simulink model "W01_Base_Map_cs"  (R2019a)
(part 2 of 32)

      settings: OpenFcn=open_system([gcb '/Actuator'],'mask')
      mask Help: eval('openHelp(230)')
      mask Display: image(imread('TextureColor.png'))
  VISUColorRegion_Lower_Body_Male_wLongCoat_1 : Subsystem  Tag=actuator/ColorRegion  Priority=0  LoadFcn=load('PrescanColorData')  mask(PreScan Sink Block: VisuTextureColor){}
      mask help:
      | The VisuTextureColor block provides a way to adapt the color of a vehicle.
      |
      | For more information, please click Help.
      settings: OpenFcn=open_system([gcb '/Actuator'],'mask')
      mask Help: eval('openHelp(230)')
      mask Display: image(imread('TextureColor.png'))
  VISUColorRegion_Lower_Body_Man_250_1 : Subsystem  Tag=actuator/ColorRegion  Priority=0  LoadFcn=load('PrescanColorData')  mask(PreScan Sink Block: VisuTextureColor){}
      mask help:
      | The VisuTextureColor block provides a way to adapt the color of a vehicle.
      |
      | For more information, please click Help.
      settings: OpenFcn=open_system([gcb '/Actuator'],'mask')
      mask Help: eval('openHelp(230)')
      mask Display: image(imread('TextureColor.png'))
  VISUColorRegion_Shoes_Boy_150_1 : Subsystem  Tag=actuator/ColorRegion  Priority=0  LoadFcn=load('PrescanColorData')  mask(PreScan Sink Block: VisuTextureColor){}
      mask help:
      | The VisuTextureColor block provides a way to adapt the color of a vehicle.
      |
      | For more information, please click Help.
      settings: OpenFcn=open_system([gcb '/Actuator'],'mask')
      mask Help: eval('openHelp(230)')
      mask Display: image(imread('TextureColor.png'))
  VISUColorRegion_Shoes_Child_Overweight_1 : Subsystem  Tag=actuator/ColorRegion  Priority=0  LoadFcn=load('PrescanColorData')  mask(PreScan Sink Block: VisuTextureColor){}
      mask help:
      | The VisuTextureColor block provides a way to adapt the color of a vehicle.
      |
      | For more information, please click Help.
      settings: OpenFcn=open_system([gcb '/Actuator'],'mask')
      mask Help: eval('openHelp(230)')
      mask Display: image(imread('TextureColor.png'))
  VISUColorRegion_Shoes_Female_Overweight_1 : Subsystem  Tag=actuator/ColorRegion  Priority=0  LoadFcn=load('PrescanColorData')  mask(PreScan Sink Block: VisuTextureColor){}
      mask help:
      | The VisuTextureColor block provides a way to adapt the color of a vehicle.
      |
      | For more information, please click Help.
      settings: OpenFcn=open_system([gcb '/Actuator'],'mask')
      mask Help: eval('openHelp(230)')
      mask Display: image(imread('TextureColor.png'))
  VISUColorRegion_Shoes_Female_Regular_1 : Subsystem  Tag=actuator/ColorRegion  Priority=0  LoadFcn=load('PrescanColorData')  mask(PreScan Sink Block: VisuTextureColor){}
      mask help:
      | The VisuTextureColor block provides a way to adapt the color of a vehicle.
      |
      | For more information, please click Help.
      settings: OpenFcn=open_system([gcb '/Actuator'],'mask')
      mask Help: eval('openHelp(230)')
      mask Display: image(imread('TextureColor.png'))
  VISUColorRegion_Shoes_Female_wBuggy_1 : Subsystem  Tag=actuator/ColorRegion  Priority=0  LoadFcn=load('PrescanColorData')  mask(PreScan Sink Block: VisuTextureColor){}
      mask help:
      | The VisuTextureColor block provides a way to adapt the color of a vehicle.
      |
      | For more information, please click Help.
      settings: OpenFcn=open_system([gcb '/Actuator'],'mask')
      mask Help: eval('openHelp(230)')
      mask Display: image(imread('TextureColor.png'))
  VISUColorRegion_Shoes_Female_wLongCoat_1 : Subsystem  Tag=actuator/ColorRegion  Priority=0  LoadFcn=load('PrescanColorData')  mask(PreScan Sink Block: VisuTextureColor){}
      mask help:
      | The VisuTextureColor block provides a way to adapt the color of a vehicle.
      |
      | For more information, please click Help.
      settings: OpenFcn=open_system([gcb '/Actuator'],'mask')
      mask Help: eval('openHelp(230)')
      mask Display: image(imread('TextureColor.png'))
  VISUColorRegion_Shoes_Female_wRaincoat_1 : Subsystem  Tag=actuator/ColorRegion  Priority=0  LoadFcn=load('PrescanColorData')  mask(PreScan Sink Block: VisuTextureColor){}
      mask help:
      | The VisuTextureColor block provides a way to adapt the color of a vehicle.
      |
      | For more information, please click Help.
      settings: OpenFcn=open_system([gcb '/Actuator'],'mask')
      mask Help: eval('openHelp(230)')
      mask Display: image(imread('TextureColor.png'))
  VISUColorRegion_Shoes_Male_200_1 : Subsystem  Tag=actuator/ColorRegion  Priority=0  LoadFcn=load('PrescanColorData')  mask(PreScan Sink Block: VisuTextureColor){}
      mask help:
      | The VisuTextureColor block provides a way to adapt the color of a vehicle.
      |
      | For more information, please click Help.
      settings: OpenFcn=open_system([gcb '/Actuator'],'mask')
      mask Help: eval('openHelp(230)')
      mask Display: image(imread('TextureColor.png'))
  VISUColorRegion_Shoes_Male_African_1 : Subsystem  Tag=actuator/ColorRegion  Priority=0  LoadFcn=load('PrescanColorData')  mask(PreScan Sink Block: VisuTextureColor){}
      mask help:
      | The VisuTextureColor block provides a way to adapt the color of a vehicle.
      |
      | For more information, please click Help.
      settings: OpenFcn=open_system([gcb '/Actuator'],'mask')
      mask Help: eval('openHelp(230)')
      mask Display: image(imread('TextureColor.png'))
  VISUColorRegion_Shoes_Male_LargeShoulderSuitcase_1 : Subsystem  Tag=actuator/ColorRegion  Priority=0  LoadFcn=load('PrescanColorData')  mask(PreScan Sink Block: VisuTextureColor){}
      mask help:
      | The VisuTextureColor block provides a way to adapt the color of a vehicle.
      |
      | For more information, please click Help.
      settings: OpenFcn=open_system([gcb '/Actuator'],'mask')
      mask Help: eval('openHelp(230)')
      mask Display: image(imread('TextureColor.png'))
  VISUColorRegion_Shoes_Male_Old_White_WithStick_1 : Subsystem  Tag=actuator/ColorRegion  Priority=0  LoadFcn=load('PrescanColorData')  mask(PreScan Sink Block: VisuTextureColor){}
      mask help:
      | The VisuTextureColor block provides a way to adapt the color of a vehicle.
      |
      | For more information, please click Help.
      settings: OpenFcn=open_system([gcb '/Actuator'],'mask')
      mask Help: eval('openHelp(230)')
      mask Display: image(imread('TextureColor.png'))
  VISUColorRegion_Shoes_Male_Old_White_WithWalkerWithWheels_1 : Subsystem  Tag=actuator/ColorRegion  Priority=0  LoadFcn=load('PrescanColorData')  mask(PreScan Sink Block: VisuTextureColor){}
      mask help:
      | The VisuTextureColor block provides a way to adapt the color of a vehicle.
      |
      | For more information, please click Help.
      settings: OpenFcn=open_system([gcb '/Actuator'],'mask')
      mask Help: eval('openHelp(230)')
      mask Display: image(imread('TextureColor.png'))
  VISUColorRegion_Shoes_Male_Overweight_1 : Subsystem  Tag=actuator/ColorRegion  Priority=0  LoadFcn=load('PrescanColorData')  mask(PreScan Sink Block: VisuTextureColor){}
      mask help:
      | The VisuTextureColor block provides a way to adapt the color of a vehicle.
      |
      | For more information, please click Help.
      settings: OpenFcn=open_system([gcb '/Actuator'],'mask')
      mask Help: eval('openHelp(230)')
      mask Display: image(imread('TextureColor.png'))
  VISUColorRegion_Shoes_Male_ShoppingBag_1 : Subsystem  Tag=actuator/ColorRegion  Priority=0  LoadFcn=load('PrescanColorData')  mask(PreScan Sink Block: VisuTextureColor){}
      mask help:
      | The VisuTextureColor block provides a way to adapt the color of a vehicle.
      |
      | For more information, please click Help.
      settings: OpenFcn=open_system([gcb '/Actuator'],'mask')
      mask Help: eval('openHelp(230)')
      mask Display: image(imread('TextureColor.png'))
  VISUColorRegion_Shoes_Male_wBackpack_1 : Subsystem  Tag=actuator/ColorRegion  Priority=0  LoadFcn=load('PrescanColorData')  mask(PreScan Sink Block: VisuTextureColor){}
      mask help:
      | The VisuTextureColor block provides a way to adapt the color of a vehicle.
      |
      | For more information, please click Help.
      settings: OpenFcn=open_system([gcb '/Actuator'],'mask')
      mask Help: eval('openHelp(230)')
      mask Display: image(imread('TextureColor.png'))
  VISUColorRegion_Shoes_Male_wLargeBackpack_1 : Subsystem  Tag=actuator/ColorRegion  Priority=0  LoadFcn=load('PrescanColorData')  mask(PreScan Sink Block: VisuTextureColor){}
      mask help:
      | The VisuTextureColor block provides a way to adapt the color of a vehicle.
      |
      | For more information, please click Help.
      settings: OpenFcn=open_system([gcb '/Actuator'],'mask')
      mask Help: eval('openHelp(230)')
      mask Display: image(imread('TextureColor.png'))
  VISUColorRegion_Shoes_Male_wLongCoat_1 : Subsystem  Tag=actuator/ColorRegion  Priority=0  LoadFcn=load('PrescanColorData')  mask(PreScan Sink Block: VisuTextureColor){}
      mask help:
      | The VisuTextureColor block provides a way to adapt the color of a vehicle.
      |
      | For more information, please click Help.
      settings: OpenFcn=open_system([gcb '/Actuator'],'mask')
      mask Help: eval('openHelp(230)')
      mask Display: image(imread('TextureColor.png'))
  VISUColorRegion_Shoes_Man_250_1 : Subsystem  Tag=actuator/ColorRegion  Priority=0  LoadFcn=load('PrescanColorData')  mask(PreScan Sink Block: VisuTextureColor){}
      mask help:
      | The VisuTextureColor block provides a way to adapt the color of a vehicle.
      |
      | For more information, please click Help.
      settings: OpenFcn=open_system([gcb '/Actuator'],'mask')
      mask Help: eval('openHelp(230)')
      mask Display: image(imread('TextureColor.png'))
  VISUColorRegion_Upper_Body_Boy_150_1 : Subsystem  Tag=actuator/ColorRegion  Priority=0  LoadFcn=load('PrescanColorData')  mask(PreScan Sink Block: VisuTextureColor){}
      mask help:
      | The VisuTextureColor block provides a way to adapt the color of a vehicle.
      |
      | For more information, please click Help.
      settings: OpenFcn=open_system([gcb '/Actuator'],'mask')
      mask Help: eval('openHelp(230)')
      mask Display: image(imread('TextureColor.png'))
  VISUColorRegion_Upper_Body_Child_Overweight_1 : Subsystem  Tag=actuator/ColorRegion  Priority=0  LoadFcn=load('PrescanColorData')  mask(PreScan Sink Block: VisuTextureColor){}
      mask help:
      | The VisuTextureColor block provides a way to adapt the color of a vehicle.
      |
      | For more information, please click Help.
      settings: OpenFcn=open_system([gcb '/Actuator'],'mask')
      mask Help: eval('openHelp(230)')
      mask Display: image(imread('TextureColor.png'))
  VISUColorRegion_Upper_Body_Female_Overweight_1 : Subsystem  Tag=actuator/ColorRegion  Priority=0  LoadFcn=load('PrescanColorData')  mask(PreScan Sink Block: VisuTextureColor){}
      mask help:
      | The VisuTextureColor block provides a way to adapt the color of a vehicle.
      |
      | For more information, please click Help.
      settings: OpenFcn=open_system([gcb '/Actuator'],'mask')
      mask Help: eval('openHelp(230)')
      mask Display: image(imread('TextureColor.png'))
  VISUColorRegion_Upper_Body_Female_Regular_1 : Subsystem  Tag=actuator/ColorRegion  Priority=0  LoadFcn=load('PrescanColorData')  mask(PreScan Sink Block: VisuTextureColor){}
      mask help:
      | The VisuTextureColor block provides a way to adapt the color of a vehicle.
      |
      | For more information, please click Help.
      settings: OpenFcn=open_system([gcb '/Actuator'],'mask')
      mask Help: eval('openHelp(230)')
      mask Display: image(imread('TextureColor.png'))
  VISUColorRegion_Upper_Body_Female_wBuggy_1 : Subsystem  Tag=actuator/ColorRegion  Priority=0  LoadFcn=load('PrescanColorData')  mask(PreScan Sink Block: VisuTextureColor){}
      mask help:
      | The VisuTextureColor block provides a way to adapt the color of a vehicle.
      |
      | For more information, please click Help.
      settings: OpenFcn=open_system([gcb '/Actuator'],'mask')
      mask Help: eval('openHelp(230)')
      mask Display: image(imread('TextureColor.png'))
  VISUColorRegion_Upper_Body_Female_wLongCoat_1 : Subsystem  Tag=actuator/ColorRegion  Priority=0  LoadFcn=load('PrescanColorData')  mask(PreScan Sink Block: VisuTextureColor){}
      mask help:
      | The VisuTextureColor block provides a way to adapt the color of a vehicle.
      |
      | For more information, please click Help.
      settings: OpenFcn=open_system([gcb '/Actuator'],'mask')
      mask Help: eval('openHelp(230)')
      mask Display: image(imread('TextureColor.png'))
  VISUColorRegion_Upper_Body_Female_wRaincoat_1 : Subsystem  Tag=actuator/ColorRegion  Priority=0  LoadFcn=load('PrescanColorData')  mask(PreScan Sink Block: VisuTextureColor){}
      mask help:
      | The VisuTextureColor block provides a way to adapt the color of a vehicle.
      |
      | For more information, please click Help.
      settings: OpenFcn=open_system([gcb '/Actuator'],'mask')
      mask Help: eval('openHelp(230)')
      mask Display: image(imread('TextureColor.png'))
  VISUColorRegion_Upper_Body_Male_200_1 : Subsystem  Tag=actuator/ColorRegion  Priority=0  LoadFcn=load('PrescanColorData')  mask(PreScan Sink Block: VisuTextureColor){}
      mask help:
      | The VisuTextureColor block provides a way to adapt the color of a vehicle.
      |
      | For more information, please click Help.
      settings: OpenFcn=open_system([gcb '/Actuator'],'mask')
      mask Help: eval('openHelp(230)')
      mask Display: image(imread('TextureColor.png'))
  VISUColorRegion_Upper_Body_Male_African_1 : Subsystem  Tag=actuator/ColorRegion  Priority=0  LoadFcn=load('PrescanColorData')  mask(PreScan Sink Block: VisuTextureColor){}
      mask help:
      | The VisuTextureColor block provides a way to adapt the color of a vehicle.
      |
      | For more information, please click Help.
      settings: OpenFcn=open_system([gcb '/Actuator'],'mask')
      mask Help: eval('openHelp(230)')
      mask Display: image(imread('TextureColor.png'))
  VISUColorRegion_Upper_Body_Male_Old_White_WithStick_1 : Subsystem  Tag=actuator/ColorRegion  Priority=0  LoadFcn=load('PrescanColorData')  mask(PreScan Sink Block: VisuTextureColor){}
      mask help:
      | The VisuTextureColor block provides a way to adapt the color of a vehicle.
      |
      | For more information, please click Help.
      settings: OpenFcn=open_system([gcb '/Actuator'],'mask')
      mask Help: eval('openHelp(230)')
      mask Display: image(imread('TextureColor.png'))
  VISUColorRegion_Upper_Body_Male_Old_White_WithWalkerWithWheels_1 : Subsystem  Tag=actuator/ColorRegion  Priority=0  LoadFcn=load('PrescanColorData')  mask(PreScan Sink Block: VisuTextureColor){}
      mask help:
      | The VisuTextureColor block provides a way to adapt the color of a vehicle.
      |
      | For more information, please click Help.
      settings: OpenFcn=open_system([gcb '/Actuator'],'mask')
      mask Help: eval('openHelp(230)')
      mask Display: image(imread('TextureColor.png'))
  VISUColorRegion_Upper_Body_Male_ShoppingBag_1 : Subsystem  Tag=actuator/ColorRegion  Priority=0  LoadFcn=load('PrescanColorData')  mask(PreScan Sink Block: VisuTextureColor){}
      mask help:
      | The VisuTextureColor block provides a way to adapt the color of a vehicle.
      |
      | For more information, please click Help.
      settings: OpenFcn=open_system([gcb '/Actuator'],'mask')
      mask Help: eval('openHelp(230)')
      mask Display: image(imread('TextureColor.png'))
  VISUColorRegion_Upper_Body_Male_wBackpack_1 : Subsystem  Tag=actuator/ColorRegion  Priority=0  LoadFcn=load('PrescanColorData')  mask(PreScan Sink Block: VisuTextureColor){}
      mask help:
      | The VisuTextureColor block provides a way to adapt the color of a vehicle.
      |
      | For more information, please click Help.
      settings: OpenFcn=open_system([gcb '/Actuator'],'mask')
      mask Help: eval('openHelp(230)')
      mask Display: image(imread('TextureColor.png'))
  VISUColorRegion_Upper_Body_Male_wLongCoat_1 : Subsystem  Tag=actuator/ColorRegion  Priority=0  LoadFcn=load('PrescanColorData')  mask(PreScan Sink Block: VisuTextureColor){}
      mask help:
      | The VisuTextureColor block provides a way to adapt the color of a vehicle.
      |
      | For more information, please click Help.
      settings: OpenFcn=open_system([gcb '/Actuator'],'mask')
      mask Help: eval('openHelp(230)')
      mask Display: image(imread('TextureColor.png'))
  VISUColorRegion_Upper_Body_Man_250_1 : Subsystem  Tag=actuator/ColorRegion  Priority=0  LoadFcn=load('PrescanColorData')  mask(PreScan Sink Block: VisuTextureColor){}
      mask help:
      | The VisuTextureColor block provides a way to adapt the color of a vehicle.
      |
      | For more information, please click Help.
      settings: OpenFcn=open_system([gcb '/Actuator'],'mask')
      mask Help: eval('openHelp(230)')
      mask Display: image(imread('TextureColor.png'))
  VISUColorRegion_Upper_body_Male_LargeShoulderSuitcase_1 : Subsystem  Tag=actuator/ColorRegion  Priority=0  LoadFcn=load('PrescanColorData')  mask(PreScan Sink Block: VisuTextureColor){}
      mask help:
      | The VisuTextureColor block provides a way to adapt the color of a vehicle.
      |
      | For more information, please click Help.
      settings: OpenFcn=open_system([gcb '/Actuator'],'mask')
      mask Help: eval('openHelp(230)')
      mask Display: image(imread('TextureColor.png'))
  VISUColorRegion_Upper_body_Male_wLargeBackpack_1 : Subsystem  Tag=actuator/ColorRegion  Priority=0  LoadFcn=load('PrescanColorData')  mask(PreScan Sink Block: VisuTextureColor){}
      mask help:
      | The VisuTextureColor block provides a way to adapt the color of a vehicle.
      |
      | For more information, please click Help.
      settings: OpenFcn=open_system([gcb '/Actuator'],'mask')
      mask Help: eval('openHelp(230)')
      mask Display: image(imread('TextureColor.png'))
  Vector Concatenate : Concatenate  Commented=on  NumInputs=3
  Volvo_XC60_1 : Subsystem  Tag=WorldObjectSubSystem  InitFcn=UniqueId = '29038';
      mask init:
      | modelPath = GenericModelHelper.getGenericModelFilePath('ModelDepo','Vehicles\Volvo_XC60\VolvoXC60.pgmb','fe213b90741b40e4bc1c1ba1f9c63fa4');imagePath = GenericModelHelper.getCompilationPicture(modelPath, 'Volvo_XC60.png');
      mask Display: image(imread(imagePath));color('white');text(0, 0, ' ID=122\n')
  Wuling_Hongguang_1 : Subsystem  Tag=WorldObjectSubSystem  InitFcn=UniqueId = '29075';
      mask init:
      | modelPath = GenericModelHelper.getGenericModelFilePath('ModelDepo','Vehicles\Wuling_Hongguang\Wuling_Hongguang.pgmb','c2d1d1bd61267082ac42dab8ff861914');imagePath = GenericModelHelper.getCompilationPicture(modelPath, 'Wuling_Hongguang.png');
      mask Display: image(imread(imagePath));color('white');text(0, 0, ' ID=151\n')
  pose_otheCar : Subsystem  Commented=on
  wires:
  From9/1 -> pose_otheCar/Enable
  Vector Concatenate/1 -> pose_otheCar/1(In1)
  Subsystem/1(Out1) -> Female_Regular_1/2(In1)
  Subsystem/2(Out2) -> Male_wLargeBackpack_1/2(In1)
  Subsystem/3(Out3) -> Male_wBackpack_1/2(In1)
  Subsystem/4(Out4) -> Male_ShoppingBag_1/2(In1)
  Subsystem/5(Out5) -> Male_LargeShoulderSuitcase_1/2(In1)
  Subsystem/6(Out6) -> Male_wLongCoat_1/2(In1)
  Subsystem/7(Out7) -> Honda_Pan_European_Motorcycle_With_Driver_1/2(In1)
  Subsystem/8(Out8) -> Sports_Bike_wDriver_1/2(In1)
  Subsystem/9(Out9) -> Tesla_Model_3_1/2(In1)
  Subsystem/10(Out10) -> Volvo_XC60_1/2(In1)
  Subsystem/11(Out11) -> Boy_150_1/2(In1)
  Subsystem/12(Out12) -> Child_Overweight_1/2(In1)
  Subsystem/13(Out13) -> Female_Overweight_1/2(In1)
  Subsystem/14(Out14) -> Female_wBuggy_1/2(In1)
  Subsystem/15(Out15) -> Female_wLongCoat_1/2(In1)
  Subsystem/16(Out16) -> Female_wRaincoat_1/2(In1)
  Subsystem/17(Out17) -> Male_African_1/2(In1)
  Subsystem/18(Out18) -> Male_Old_White_WithStick_1/2(In1)
  Subsystem/19(Out19) -> Male_Overweight_1/2(In1)
  Subsystem/20(Out20) -> Male_wSuit_1/2(In1)
  Subsystem/21(Out21) -> Male_200_1/2(In1)
  Subsystem/22(Out22) -> Man_250_1/2(In1)
  Subsystem/23(Out23) -> Male_Old_White_WithWalker_1/2(In1)
  Subsystem/24(Out24) -> Male_Old_White_WithWalkerWithWheels_1/2(In1)
  Subsystem/25(Out25) -> Audi_A3_1/2(In1)
  Subsystem/26(Out26) -> Audi_A8_Sedan_2/2(In1)
  Subsystem/27(Out27) -> BMW_Z3_Convertible_1/2(In1)
  Subsystem/28(Out28) -> Citroen_C3_Hatchback_2/2(In1)
  Subsystem/29(Out29) -> Fiat_Bravo_Hatchback_1/2(In1)
  Subsystem/30(Out30) -> Ford_Fiesta_Hatchback_2/2(In1)
  Subsystem/31(Out31) -> Ford_Focus_Stationwagon_1/2(In1)
  Subsystem/32(Out32) -> Lexus_GS_450h_F_Sport_Sedan_1/2(In1)
  Subsystem/33(Out33) -> Lexus_LS_600h_F_Sport_1/2(In1)
  Subsystem/34(Out34) -> Mazda_RX8_Coupe_1/2(In1)
  Subsystem/35(Out35) -> Roewe_550_S_Sedan_1/2(In1)
  Subsystem/36(Out36) -> Toyota_Previa_MPV_1/2(In1)
  Subsystem/37(Out37) -> Toyota_Prius_Sedan_1/2(In1)
  Subsystem/38(Out38) -> Toyota_Yaris_Hatchback_1/2(In1)
  Subsystem/39(Out39) -> Wuling_Hongguang_1/2(In1)
  Subsystem/40(Out40) -> Toyota_Yaris_Hatchback_2/2(In1)
  Subsystem/41(Out41) -> Citroen_C3_Hatchback_3/2(In1)
  Subsystem/42(Out42) -> Audi_A3_2/2(In1)
  Subsystem/43(Out43) -> Sports_Bike_wDriver_2/2(In1)
  Subsystem/44(Out44) -> Sports_Bike_wDriver_3/2(In1)
  Subsystem/45(Out45) -> Honda_Pan_European_Motorcycle_With_Driver_2/2(In1)
  Subsystem/46(Out46) -> Male_CyclingCyclist_1/2(In1)
  Subsystem/47(Out47) -> Male_CyclingCyclist_2/2(In1)
  Subsystem/48(Out48) -> Male_CyclingCyclist_3/2(In1)
  Subsystem/49(Out49) -> Male_CyclingCyclist_4/2(In1)
  Subsystem/50(Out50) -> Male_CyclingCyclist_5/2(In1)
  Subsystem/51(Out51) -> Male_CyclingCyclist_6/2(In1)
  Subsystem/52(Out52) -> Male_CyclingCyclist_7/2(In1)
  Subsystem/53(Out53) -> Male_CyclingCyclist_8/2(In1)
  Subsystem/54(Out54) -> Male_CyclingCyclist_9/2(In1)
  Subsystem/55(Out55) -> Male_CyclingCyclist_10/2(In1)
  BMW_X5_SUV_1/1(STATE_BMW_X5_SUV_1_bus) -> STATE_BMW_X5_SUV_1_bus/1(STATE_BMW_X5_SUV_1_bus)
  SELF_BMW_X5_SUV_1/1(SELF_BMW_X5_SUV_1) -> BMW_X5_SUV_1/1(SELF_BMW_X5_SUV_1)
  Radar_1/1(Radar_1) -> BMW_X5_SUV_1/2(Radar_1)
  PointCloudSensor_1/1(PointCloudSensor_1) -> BMW_X5_SUV_1/3(PointCloudSensor_1)
  PointCloudSensor_2/1(PointCloudSensor_2) -> BMW_X5_SUV_1/4(PointCloudSensor_2)
  PointCloudSensor_3/1(PointCloudSensor_3) -> BMW_X5_SUV_1/5(PointCloudSensor_3)
  PointCloudSensor_4/1(PointCloudSensor_4) -> BMW_X5_SUV_1/6(PointCloudSensor_4)
  Camera_1/1(Camera_1) -> BMW_X5_SUV_1/7(Camera_1)
  Camera_tl/1(Camera_tl) -> BMW_X5_SUV_1/8(Camera_tl)
  Camera_2/1(Camera_2) -> BMW_X5_SUV_1/9(Camera_2)
  TrafficLightRoadSideNL_1/1(TrafficLightRoadSideNL_1_Red) -> TrafficLightRoadSideNL_1_Red/1(TrafficLightRoadSideNL_1_Red)
  TrafficLightRoadSideNL_1/2(TrafficLightRoadSideNL_1_Orange) -> TrafficLightRoadSideNL_1_Orange/1(TrafficLightRoadSideNL_1_Orange)
  TrafficLightRoadSideNL_1/3(TrafficLightRoadSideNL_1_Green) -> TrafficLightRoadSideNL_1_Green/1(TrafficLightRoadSideNL_1_Green)
  TrafficLightRoadSideNL_2/1(TrafficLightRoadSideNL_2_Red) -> TrafficLightRoadSideNL_2_Red/1(TrafficLightRoadSideNL_2_Red)
  TrafficLightRoadSideNL_2/2(TrafficLightRoadSideNL_2_Orange) -> TrafficLightRoadSideNL_2_Orange/1(TrafficLightRoadSideNL_2_Orange)
  TrafficLightRoadSideNL_2/3(TrafficLightRoadSideNL_2_Green) -> TrafficLightRoadSideNL_2_Green/1(TrafficLightRoadSideNL_2_Green)
  TrafficLightRoadSideNL_3/1(TrafficLightRoadSideNL_3_Red) -> TrafficLightRoadSideNL_3_Red/1(TrafficLightRoadSideNL_3_Red)
  TrafficLightRoadSideNL_3/2(TrafficLightRoadSideNL_3_Orange) -> TrafficLightRoadSideNL_3_Orange/1(TrafficLightRoadSideNL_3_Orange)
  TrafficLightRoadSideNL_3/3(TrafficLightRoadSideNL_3_Green) -> TrafficLightRoadSideNL_3_Green/1(TrafficLightRoadSideNL_3_Green)
  TrafficLightRoadSideNL_4/1(TrafficLightRoadSideNL_4_Red) -> TrafficLightRoadSideNL_4_Red/1(TrafficLightRoadSideNL_4_Red)
  TrafficLightRoadSideNL_4/2(TrafficLightRoadSideNL_4_Orange) -> TrafficLightRoadSideNL_4_Orange/1(TrafficLightRoadSideNL_4_Orange)
  TrafficLightRoadSideNL_4/3(TrafficLightRoadSideNL_4_Green) -> TrafficLightRoadSideNL_4_Green/1(TrafficLightRoadSideNL_4_Green)
  TrafficLightRoadSideNL_5/1(TrafficLightRoadSideNL_5_Red) -> TrafficLightRoadSideNL_5_Red/1(TrafficLightRoadSideNL_5_Red)
  TrafficLightRoadSideNL_5/2(TrafficLightRoadSideNL_5_Orange) -> TrafficLightRoadSideNL_5_Orange/1(TrafficLightRoadSideNL_5_Orange)
  TrafficLightRoadSideNL_5/3(TrafficLightRoadSideNL_5_Green) -> TrafficLightRoadSideNL_5_Green/1(TrafficLightRoadSideNL_5_Green)
  TrafficLightRoadSideNL_7/1(TrafficLightRoadSideNL_7_Red) -> TrafficLightRoadSideNL_7_Red/1(TrafficLightRoadSideNL_7_Red)
  TrafficLightRoadSideNL_7/2(TrafficLightRoadSideNL_7_Orange) -> TrafficLightRoadSideNL_7_Orange/1(TrafficLightRoadSideNL_7_Orange)
  TrafficLightRoadSideNL_7/3(TrafficLightRoadSideNL_7_Green) -> TrafficLightRoadSideNL_7_Green/1(TrafficLightRoadSideNL_7_Green)
  TrafficLightRoadSideNL_8/1(TrafficLightRoadSideNL_8_Red) -> TrafficLightRoadSideNL_8_Red/1(TrafficLightRoadSideNL_8_Red)
  TrafficLightRoadSideNL_8/2(TrafficLightRoadSideNL_8_Orange) -> TrafficLightRoadSideNL_8_Orange/1(TrafficLightRoadSideNL_8_Orange)
  TrafficLightRoadSideNL_8/3(TrafficLightRoadSideNL_8_Green) -> TrafficLightRoadSideNL_8_Green/1(TrafficLightRoadSideNL_8_Green)
  TrafficLightRoadSideNL_6/1(TrafficLightRoadSideNL_6_Red) -> TrafficLightRoadSideNL_6_Red/1(TrafficLightRoadSideNL_6_Red)
  TrafficLightRoadSideNL_6/2(TrafficLightRoadSideNL_6_Orange) -> TrafficLightRoadSideNL_6_Orange/1(TrafficLightRoadSideNL_6_Orange)
  TrafficLightRoadSideNL_6/3(TrafficLightRoadSideNL_6_Green) -> TrafficLightRoadSideNL_6_Green/1(TrafficLightRoadSideNL_6_Green)
  Female_Regular_1/1(STATE_Female_Regular_1_bus) -> STATE_Female_Regular_1_bus/1(STATE_Female_Regular_1_bus)
  Female_Regular_1/2(ANIM_Female_Regular_1) -> ANIM_Female_Regular_1/1(ANIM_Female_Regular_1)
  SELF_Female_Regular_1/1(SELF_Female_Regular_1) -> Female_Regular_1/1(SELF_Female_Regular_1)
  Female_Regular_1/3(VISUColorRegion_Upper_Body_Female_Regular_1) -> VISUColorRegion_Upper_Body_Female_Regular_1/1(VISUColorRegion_Upper_Body_Female_Regular_1)
  Female_Regular_1/4(VISUColorRegion_Lower_Body_Female_Regular_1) -> VISUColorRegion_Lower_Body_Female_Regular_1/1(VISUColorRegion_Lower_Body_Female_Regular_1)
  Female_Regular_1/5(VISUColorRegion_Shoes_Female_Regular_1) -> VISUColorRegion_Shoes_Female_Regular_1/1(VISUColorRegion_Shoes_Female_Regular_1)
  Male_wLargeBackpack_1/1(STATE_Male_wLargeBackpack_1_bus) -> STATE_Male_wLargeBackpack_1_bus/1(STATE_Male_wLargeBackpack_1_bus)
  Male_wLargeBackpack_1/2(ANIM_Male_wLargeBackpack_1) -> ANIM_Male_wLargeBackpack_1/1(ANIM_Male_wLargeBackpack_1)
  SELF_Male_wLargeBackpack_1/1(SELF_Male_wLargeBackpack_1) -> Male_wLargeBackpack_1/1(SELF_Male_wLargeBackpack_1)
  Male_wLargeBackpack_1/3(VISUColorRegion_Upper_body_Male_wLargeBackpack_1) -> VISUColorRegion_Upper_body_Male_wLargeBackpack_1/1(VISUColorRegion_Upper_body_Male_wLargeBackpack_1)
  Male_wLargeBackpack_1/4(VISUColorRegion_Lower_Body_Male_wLargeBackpack_1) -> VISUColorRegion_Lower_Body_Male_wLargeBackpack_1/1(VISUColorRegion_Lower_Body_Male_wLargeBackpack_1)
  Male_wLargeBackpack_1/5(VISUColorRegion_Shoes_Male_wLargeBackpack_1) -> VISUColorRegion_Shoes_Male_wLargeBackpack_1/1(VISUColorRegion_Shoes_Male_wLargeBackpack_1)
  Male_wLargeBackpack_1/6(VISUColorRegion_Bag_Male_wLargeBackpack_1) -> VISUColorRegion_Bag_Male_wLargeBackpack_1/1(VISUColorRegion_Bag_Male_wLargeBackpack_1)
  Male_wBackpack_1/1(STATE_Male_wBackpack_1_bus) -> STATE_Male_wBackpack_1_bus/1(STATE_Male_wBackpack_1_bus)
  Male_wBackpack_1/2(ANIM_Male_wBackpack_1) -> ANIM_Male_wBackpack_1/1(ANIM_Male_wBackpack_1)
  SELF_Male_wBackpack_1/1(SELF_Male_wBackpack_1) -> Male_wBackpack_1/1(SELF_Male_wBackpack_1)
  Male_wBackpack_1/3(VISUColorRegion_Upper_Body_Male_wBackpack_1) -> VISUColorRegion_Upper_Body_Male_wBackpack_1/1(VISUColorRegion_Upper_Body_Male_wBackpack_1)
  Male_wBackpack_1/4(VISUColorRegion_Lower_Body_Male_wBackpack_1) -> VISUColorRegion_Lower_Body_Male_wBackpack_1/1(VISUColorRegion_Lower_Body_Male_wBackpack_1)
  Male_wBackpack_1/5(VISUColorRegion_Shoes_Male_wBackpack_1) -> VISUColorRegion_Shoes_Male_wBackpack_1/1(VISUColorRegion_Shoes_Male_wBackpack_1)
  Male_ShoppingBag_1/1(STATE_Male_ShoppingBag_1_bus) -> STATE_Male_ShoppingBag_1_bus/1(STATE_Male_ShoppingBag_1_bus)
  Male_ShoppingBag_1/2(ANIM_Male_ShoppingBag_1) -> ANIM_Male_ShoppingBag_1/1(ANIM_Male_ShoppingBag_1)
  SELF_Male_ShoppingBag_1/1(SELF_Male_ShoppingBag_1) -> Male_ShoppingBag_1/1(SELF_Male_ShoppingBag_1)
  Male_ShoppingBag_1/3(VISUColorRegion_Upper_Body_Male_ShoppingBag_1) -> VISUColorRegion_Upper_Body_Male_ShoppingBag_1/1(VISUColorRegion_Upper_Body_Male_ShoppingBag_1)
  Male_ShoppingBag_1/4(VISUColorRegion_Lower_Body_Male_ShoppingBag_1) -> VISUColorRegion_Lower_Body_Male_ShoppingBag_1/1(VISUColorRegion_Lower_Body_Male_ShoppingBag_1)
  Male_ShoppingBag_1/5(VISUColorRegion_Shoes_Male_ShoppingBag_1) -> VISUColorRegion_Shoes_Male_ShoppingBag_1/1(VISUColorRegion_Shoes_Male_ShoppingBag_1)
  Male_ShoppingBag_1/6(VISUColorRegion_Bag_Male_ShoppingBag_1) -> VISUColorRegion_Bag_Male_ShoppingBag_1/1(VISUColorRegion_Bag_Male_ShoppingBag_1)
  Male_LargeShoulderSuitcase_1/1(STATE_Male_LargeShoulderSuitcase_1_bus) -> STATE_Male_LargeShoulderSuitcase_1_bus/1(STATE_Male_LargeShoulderSuitcase_1_bus)
  Male_LargeShoulderSuitcase_1/2(ANIM_Male_LargeShoulderSuitcase_1) -> ANIM_Male_LargeShoulderSuitcase_1/1(ANIM_Male_LargeShoulderSuitcase_1)
  SELF_Male_LargeShoulderSuitcase_1/1(SELF_Male_LargeShoulderSuitcase_1) -> Male_LargeShoulderSuitcase_1/1(SELF_Male_LargeShoulderSuitcase_1)
  Male_LargeShoulderSuitcase_1/3(VISUColorRegion_Upper_body_Male_LargeShoulderSuitcase_1) -> VISUColorRegion_Upper_body_Male_LargeShoulderSuitcase_1/1(VISUColorRegion_Upper_body_Male_LargeShoulderSuitcase_1)
  Male_LargeShoulderSuitcase_1/4(VISUColorRegion_Lower_Body_Male_LargeShoulderSuitcase_1) -> VISUColorRegion_Lower_Body_Male_LargeShoulderSuitcase_1/1(VISUColorRegion_Lower_Body_Male_LargeShoulderSuitcase_1)
  Male_LargeShoulderSuitcase_1/5(VISUColorRegion_Shoes_Male_LargeShoulderSuitcase_1) -> VISUColorRegion_Shoes_Male_LargeShoulderSuitcase_1/1(VISUColorRegion_Shoes_Male_LargeShoulderSuitcase_1)
  Male_LargeShoulderSuitcase_1/6(VISUColorRegion_Bag_Male_LargeShoulderSuitcase_1) -> VISUColorRegion_Bag_Male_LargeShoulderSuitcase_1/1(VISUColorRegion_Bag_Male_LargeShoulderSuitcase_1)
  Male_wLongCoat_1/1(STATE_Male_wLongCoat_1_bus) -> STATE_Male_wLongCoat_1_bus/1(STATE_Male_wLongCoat_1_bus)
  Male_wLongCoat_1/2(ANIM_Male_wLongCoat_1) -> ANIM_Male_wLongCoat_1/1(ANIM_Male_wLongCoat_1)
  SELF_Male_wLongCoat_1/1(SELF_Male_wLongCoat_1) -> Male_wLongCoat_1/1(SELF_Male_wLongCoat_1)
  Male_wLongCoat_1/3(VISUColorRegion_Upper_Body_Male_wLongCoat_1) -> VISUColorRegion_Upper_Body_Male_wLongCoat_1/1(VISUColorRegion_Upper_Body_Male_wLongCoat_1)
  Male_wLongCoat_1/4(VISUColorRegion_Coat_Male_wLongCoat_1) -> VISUColorRegion_Coat_Male_wLongCoat_1/1(VISUColorRegion_Coat_Male_wLongCoat_1)
  Male_wLongCoat_1/5(VISUColorRegion_Lower_Body_Male_wLongCoat_1) -> VISUColorRegion_Lower_Body_Male_wLongCoat_1/1(VISUColorRegion_Lower_Body_Male_wLongCoat_1)
  Male_wLongCoat_1/6(VISUColorRegion_Shoes_Male_wLongCoat_1) -> VISUColorRegion_Shoes_Male_wLongCoat_1/1(VISUColorRegion_Shoes_Male_wLongCoat_1)
  Honda_Pan_European_Motorcycle_With_Driver_1/1(STATE_Honda_Pan_European_Motorcycle_With_Driver_1_bus) -> STATE_Honda_Pan_European_Motorcycle_With_Driver_1_bus/1(STATE_Honda_Pan_European_Motorcycle_With_Driver_1_bus)
  SELF_Honda_Pan_European_Motorcycle_With_Driver_1/1(SELF_Honda_Pan_European_Motorcycle_With_Driver_1) -> Honda_Pan_European_Motorcycle_With_Driver_1/1(SELF_Honda_Pan_European_Motorcycle_With_Driver_1)
  Sports_Bike_wDriver_1/1(STATE_Sports_Bike_wDriver_1_bus) -> STATE_Sports_Bike_wDriver_1_bus/1(STATE_Sports_Bike_wDriver_1_bus)
  SELF_Sports_Bike_wDriver_1/1(SELF_Sports_Bike_wDriver_1) -> Sports_Bike_wDriver_1/1(SELF_Sports_Bike_wDriver_1)
  Tesla_Model_3_1/1(STATE_Tesla_Model_3_1_bus) -> STATE_Tesla_Model_3_1_bus/1(STATE_Tesla_Model_3_1_bus)
  SELF_Tesla_Model_3_1/1(SELF_Tesla_Model_3_1) -> Tesla_Model_3_1/1(SELF_Tesla_Model_3_1)
  Volvo_XC60_1/1(STATE_Volvo_XC60_1_bus) -> STATE_Volvo_XC60_1_bus/1(STATE_Volvo_XC60_1_bus)
  SELF_Volvo_XC60_1/1(SELF_Volvo_XC60_1) -> Volvo_XC60_1/1(SELF_Volvo_XC60_1)
  Boy_150_1/1(STATE_Boy_150_1_bus) -> STATE_Boy_150_1_bus/1(STATE_Boy_150_1_bus)
  Boy_150_1/2(ANIM_Boy_150_1) -> ANIM_Boy_150_1/1(ANIM_Boy_150_1)
  SELF_Boy_150_1/1(SELF_Boy_150_1) -> Boy_150_1/1(SELF_Boy_150_1)
  Boy_150_1/3(VISUColorRegion_Upper_Body_Boy_150_1) -> VISUColorRegion_Upper_Body_Boy_150_1/1(VISUColorRegion_Upper_Body_Boy_150_1)
  Boy_150_1/4(VISUColorRegion_Lower_Body_Boy_150_1) -> VISUColorRegion_Lower_Body_Boy_150_1/1(VISUColorRegion_Lower_Body_Boy_150_1)
  Boy_150_1/5(VISUColorRegion_Shoes_Boy_150_1) -> VISUColorRegion_Shoes_Boy_150_1/1(VISUColorRegion_Shoes_Boy_150_1)
  Child_Overweight_1/1(STATE_Child_Overweight_1_bus) -> STATE_Child_Overweight_1_bus/1(STATE_Child_Overweight_1_bus)
  Child_Overweight_1/2(ANIM_Child_Overweight_1) -> ANIM_Child_Overweight_1/1(ANIM_Child_Overweight_1)
  SELF_Child_Overweight_1/1(SELF_Child_Overweight_1) -> Child_Overweight_1/1(SELF_Child_Overweight_1)
  Child_Overweight_1/3(VISUColorRegion_Upper_Body_Child_Overweight_1) -> VISUColorRegion_Upper_Body_Child_Overweight_1/1(VISUColorRegion_Upper_Body_Child_Overweight_1)
  Child_Overweight_1/4(VISUColorRegion_Lower_Body_Child_Overweight_1) -> VISUColorRegion_Lower_Body_Child_Overweight_1/1(VISUColorRegion_Lower_Body_Child_Overweight_1)
  Child_Overweight_1/5(VISUColorRegion_Shoes_Child_Overweight_1) -> VISUColorRegion_Shoes_Child_Overweight_1/1(VISUColorRegion_Shoes_Child_Overweight_1)
  Female_Overweight_1/1(STATE_Female_Overweight_1_bus) -> STATE_Female_Overweight_1_bus/1(STATE_Female_Overweight_1_bus)
  Female_Overweight_1/2(ANIM_Female_Overweight_1) -> ANIM_Female_Overweight_1/1(ANIM_Female_Overweight_1)
  SELF_Female_Overweight_1/1(SELF_Female_Overweight_1) -> Female_Overweight_1/1(SELF_Female_Overweight_1)
  Female_Overweight_1/3(VISUColorRegion_Upper_Body_Female_Overweight_1) -> VISUColorRegion_Upper_Body_Female_Overweight_1/1(VISUColorRegion_Upper_Body_Female_Overweight_1)
  Female_Overweight_1/4(VISUColorRegion_Lower_Body_Female_Overweight_1) -> VISUColorRegion_Lower_Body_Female_Overweight_1/1(VISUColorRegion_Lower_Body_Female_Overweight_1)
  Female_Overweight_1/5(VISUColorRegion_Shoes_Female_Overweight_1) -> VISUColorRegion_Shoes_Female_Overweight_1/1(VISUColorRegion_Shoes_Female_Overweight_1)
  Female_wBuggy_1/1(STATE_Female_wBuggy_1_bus) -> STATE_Female_wBuggy_1_bus/1(STATE_Female_wBuggy_1_bus)
  Female_wBuggy_1/2(ANIM_Female_wBuggy_1) -> ANIM_Female_wBuggy_1/1(ANIM_Female_wBuggy_1)
  SELF_Female_wBuggy_1/1(SELF_Female_wBuggy_1) -> Female_wBuggy_1/1(SELF_Female_wBuggy_1)
  Female_wBuggy_1/3(VISUColorRegion_Upper_Body_Female_wBuggy_1) -> VISUColorRegion_Upper_Body_Female_wBuggy_1/1(VISUColorRegion_Upper_Body_Female_wBuggy_1)
  Female_wBuggy_1/4(VISUColorRegion_Lower_Body_Female_wBuggy_1) -> VISUColorRegion_Lower_Body_Female_wBuggy_1/1(VISUColorRegion_Lower_Body_Female_wBuggy_1)
  Female_wBuggy_1/5(VISUColorRegion_Shoes_Female_wBuggy_1) -> VISUColorRegion_Shoes_Female_wBuggy_1/1(VISUColorRegion_Shoes_Female_wBuggy_1)
  Female_wLongCoat_1/1(STATE_Female_wLongCoat_1_bus) -> STATE_Female_wLongCoat_1_bus/1(STATE_Female_wLongCoat_1_bus)
  Female_wLongCoat_1/2(ANIM_Female_wLongCoat_1) -> ANIM_Female_wLongCoat_1/1(ANIM_Female_wLongCoat_1)
  SELF_Female_wLongCoat_1/1(SELF_Female_wLongCoat_1) -> Female_wLongCoat_1/1(SELF_Female_wLongCoat_1)
  Female_wLongCoat_1/3(VISUColorRegion_Upper_Body_Female_wLongCoat_1) -> VISUColorRegion_Upper_Body_Female_wLongCoat_1/1(VISUColorRegion_Upper_Body_Female_wLongCoat_1)
  Female_wLongCoat_1/4(VISUColorRegion_Lower_Body_Female_wLongCoat_1) -> VISUColorRegion_Lower_Body_Female_wLongCoat_1/1(VISUColorRegion_Lower_Body_Female_wLongCoat_1)
  Female_wLongCoat_1/5(VISUColorRegion_Shoes_Female_wLongCoat_1) -> VISUColorRegion_Shoes_Female_wLongCoat_1/1(VISUColorRegion_Shoes_Female_wLongCoat_1)
  Female_wRaincoat_1/1(STATE_Female_wRaincoat_1_bus) -> STATE_Female_wRaincoat_1_bus/1(STATE_Female_wRaincoat_1_bus)
  Female_wRaincoat_1/2(ANIM_Female_wRaincoat_1) -> ANIM_Female_wRaincoat_1/1(ANIM_Female_wRaincoat_1)
  SELF_Female_wRaincoat_1/1(SELF_Female_wRaincoat_1) -> Female_wRaincoat_1/1(SELF_Female_wRaincoat_1)
  Female_wRaincoat_1/3(VISUColorRegion_Upper_Body_Female_wRaincoat_1) -> VISUColorRegion_Upper_Body_Female_wRaincoat_1/1(VISUColorRegion_Upper_Body_Female_wRaincoat_1)
  Female_wRaincoat_1/4(VISUColorRegion_Lower_Body_Female_wRaincoat_1) -> VISUColorRegion_Lower_Body_Female_wRaincoat_1/1(VISUColorRegion_Lower_Body_Female_wRaincoat_1)
  Female_wRaincoat_1/5(VISUColorRegion_Shoes_Female_wRaincoat_1) -> VISUColorRegion_Shoes_Female_wRaincoat_1/1(VISUColorRegion_Shoes_Female_wRaincoat_1)
  Male_African_1/1(STATE_Male_African_1_bus) -> STATE_Male_African_1_bus/1(STATE_Male_African_1_bus)
  Male_African_1/2(ANIM_Male_African_1) -> ANIM_Male_African_1/1(ANIM_Male_African_1)
  SELF_Male_African_1/1(SELF_Male_African_1) -> Male_African_1/1(SELF_Male_African_1)
  Male_African_1/3(VISUColorRegion_Upper_Body_Male_African_1) -> VISUColorRegion_Upper_Body_Male_African_1/1(VISUColorRegion_Upper_Body_Male_African_1)
  Male_African_1/4(VISUColorRegion_Lower_Body_Male_African_1) -> VISUColorRegion_Lower_Body_Male_African_1/1(VISUColorRegion_Lower_Body_Male_African_1)
  Male_African_1/5(VISUColorRegion_Shoes_Male_African_1) -> VISUColorRegion_Shoes_Male_African_1/1(VISUColorRegion_Shoes_Male_African_1)
  Male_Old_White_WithStick_1/1(STATE_Male_Old_White_WithStick_1_bus) -> STATE_Male_Old_White_WithStick_1_bus/1(STATE_Male_Old_White_WithStick_1_bus)
  SELF_Male_Old_White_WithStick_1/1(SELF_Male_Old_White_WithStick_1) -> Male_Old_White_WithStick_1/1(SELF_Male_Old_White_WithStick_1)
  Male_Old_White_WithStick_1/2(VISUColorRegion_Upper_Body_Male_Old_White_WithStick_1) -> VISUColorRegion_Upper_Body_Male_Old_White_WithStick_1/1(VISUColorRegion_Upper_Body_Male_Old_White_WithStick_1)
  Male_Old_White_WithStick_1/3(VISUColorRegion_Lower_Body_Male_Old_White_WithStick_1) -> VISUColorRegion_Lower_Body_Male_Old_White_WithStick_1/1(VISUColorRegion_Lower_Body_Male_Old_White_WithStick_1)
  Male_Old_White_WithStick_1/4(VISUColorRegion_Shoes_Male_Old_White_WithStick_1) -> VISUColorRegion_Shoes_Male_Old_White_WithStick_1/1(VISUColorRegion_Shoes_Male_Old_White_WithStick_1)
  Male_Overweight_1/1(STATE_Male_Overweight_1_bus) -> STATE_Male_Overweight_1_bus/1(STATE_Male_Overweight_1_bus)
  Male_Overweight_1/2(ANIM_Male_Overweight_1) -> ANIM_Male_Overweight_1/1(ANIM_Male_Overweight_1)
  SELF_Male_Overweight_1/1(SELF_Male_Overweight_1) -> Male_Overweight_1/1(SELF_Male_Overweight_1)
  Male_Overweight_1/3(VISUColorRegion_Lower_Body_Male_Overweight_1) -> VISUColorRegion_Lower_Body_Male_Overweight_1/1(VISUColorRegion_Lower_Body_Male_Overweight_1)
  Male_Overweight_1/4(VISUColorRegion_Shoes_Male_Overweight_1) -> VISUColorRegion_Shoes_Male_Overweight_1/1(VISUColorRegion_Shoes_Male_Overweight_1)
  Male_wSuit_1/1(STATE_Male_wSuit_1_bus) -> STATE_Male_wSuit_1_bus/1(STATE_Male_wSuit_1_bus)
  Male_wSuit_1/2(ANIM_Male_wSuit_1) -> ANIM_Male_wSuit_1/1(ANIM_Male_wSuit_1)
  SELF_Male_wSuit_1/1(SELF_Male_wSuit_1) -> Male_wSuit_1/1(SELF_Male_wSuit_1)
  Male_200_1/1(STATE_Male_200_1_bus) -> STATE_Male_200_1_bus/1(STATE_Male_200_1_bus)
  Male_200_1/2(ANIM_Male_200_1) -> ANIM_Male_200_1/1(ANIM_Male_200_1)
  SELF_Male_200_1/1(SELF_Male_200_1) -> Male_200_1/1(SELF_Male_200_1)
  Male_200_1/3(VISUColorRegion_Upper_Body_Male_200_1) -> VISUColorRegion_Upper_Body_Male_200_1/1(VISUColorRegion_Upper_Body_Male_200_1)
  Male_200_1/4(VISUColorRegion_Lower_Body_Male_200_1) -> VISUColorRegion_Lower_Body_Male_200_1/1(VISUColorRegion_Lower_Body_Male_200_1)
  Male_200_1/5(VISUColorRegion_Shoes_Male_200_1) -> VISUColorRegion_Shoes_Male_200_1/1(VISUColorRegion_Shoes_Male_200_1)
  Man_250_1/1(STATE_Man_250_1_bus) -> STATE_Man_250_1_bus/1(STATE_Man_250_1_bus)
  Man_250_1/2(ANIM_Man_250_1) -> ANIM_Man_250_1/1(ANIM_Man_250_1)
  SELF_Man_250_1/1(SELF_Man_250_1) -> Man_250_1/1(SELF_Man_250_1)
  Man_250_1/3(VISUColorRegion_Upper_Body_Man_250_1) -> VISUColorRegion_Upper_Body_Man_250_1/1(VISUColorRegion_Upper_Body_Man_250_1)
  Man_250_1/4(VISUColorRegion_Lower_Body_Man_250_1) -> VISUColorRegion_Lower_Body_Man_250_1/1(VISUColorRegion_Lower_Body_Man_250_1)
  Man_250_1/5(VISUColorRegion_Shoes_Man_250_1) -> VISUColorRegion_Shoes_Man_250_1/1(VISUColorRegion_Shoes_Man_250_1)
  Male_Old_White_WithWalker_1/1(STATE_Male_Old_White_WithWalker_1_bus) -> STATE_Male_Old_White_WithWalker_1_bus/1(STATE_Male_Old_White_WithWalker_1_bus)
  SELF_Male_Old_White_WithWalker_1/1(SELF_Male_Old_White_WithWalker_1) -> Male_Old_White_WithWalker_1/1(SELF_Male_Old_White_WithWalker_1)
  Male_Old_White_WithWalkerWithWheels_1/1(STATE_Male_Old_White_WithWalkerWithWheels_1_bus) -> STATE_Male_Old_White_WithWalkerWithWheels_1_bus/1(STATE_Male_Old_White_WithWalkerWithWheels_1_bus)
  SELF_Male_Old_White_WithWalkerWithWheels_1/1(SELF_Male_Old_White_WithWalkerWithWheels_1) -> Male_Old_White_WithWalkerWithWheels_1/1(SELF_Male_Old_White_WithWalkerWithWheels_1)
  Male_Old_White_WithWalkerWithWheels_1/2(VISUColorRegion_Upper_Body_Male_Old_White_WithWalkerWithWheels_1) -> VISUColorRegion_Upper_Body_Male_Old_White_WithWalkerWithWheels_1/1(VISUColorRegion_Upper_Body_Male_Old_White_WithWalkerWithWheels_1)
  Male_Old_White_WithWalkerWithWheels_1/3(VISUColorRegion_Lower_Body_Male_Old_White_WithWalkerWithWheels_1) -> VISUColorRegion_Lower_Body_Male_Old_White_WithWalkerWithWheels_1/1(VISUColorRegion_Lower_Body_Male_Old_White_WithWalkerWithWheels_1)
  Male_Old_White_WithWalkerWithWheels_1/4(VISUColorRegion_Shoes_Male_Old_White_WithWalkerWithWheels_1) -> VISUColorRegion_Shoes_Male_Old_White_WithWalkerWithWheels_1/1(VISUColorRegion_Shoes_Male_Old_White_WithWalkerWithWheels_1)
  Audi_A3_1/1(STATE_Audi_A3_1_bus) -> STATE_Audi_A3_1_bus/1(STATE_Audi_A3_1_bus)
  SELF_Audi_A3_1/1(SELF_Audi_A3_1) -> Audi_A3_1/1(SELF_Audi_A3_1)
  Audi_A8_Sedan_2/1(STATE_Audi_A8_Sedan_2_bus) -> STATE_Audi_A8_Sedan_2_bus/1(STATE_Audi_A8_Sedan_2_bus)
  SELF_Audi_A8_Sedan_2/1(SELF_Audi_A8_Sedan_2) -> Audi_A8_Sedan_2/1(SELF_Audi_A8_Sedan_2)
  BMW_Z3_Convertible_1/1(STATE_BMW_Z3_Convertible_1_bus) -> STATE_BMW_Z3_Convertible_1_bus/1(STATE_BMW_Z3_Convertible_1_bus)
  SELF_BMW_Z3_Convertible_1/1(SELF_BMW_Z3_Convertible_1) -> BMW_Z3_Convertible_1/1(SELF_BMW_Z3_Convertible_1)
  Citroen_C3_Hatchback_2/1(STATE_Citroen_C3_Hatchback_2_bus) -> STATE_Citroen_C3_Hatchback_2_bus/1(STATE_Citroen_C3_Hatchback_2_bus)
  SELF_Citroen_C3_Hatchback_2/1(SELF_Citroen_C3_Hatchback_2) -> Citroen_C3_Hatchback_2/1(SELF_Citroen_C3_Hatchback_2)
  Fiat_Bravo_Hatchback_1/1(STATE_Fiat_Bravo_Hatchback_1_bus) -> STATE_Fiat_Bravo_Hatchback_1_bus/1(STATE_Fiat_Bravo_Hatchback_1_bus)
  SELF_Fiat_Bravo_Hatchback_1/1(SELF_Fiat_Bravo_Hatchback_1) -> Fiat_Bravo_Hatchback_1/1(SELF_Fiat_Bravo_Hatchback_1)
  Ford_Fiesta_Hatchback_2/1(STATE_Ford_Fiesta_Hatchback_2_bus) -> STATE_Ford_Fiesta_Hatchback_2_bus/1(STATE_Ford_Fiesta_Hatchback_2_bus)
  SELF_Ford_Fiesta_Hatchback_2/1(SELF_Ford_Fiesta_Hatchback_2) -> Ford_Fiesta_Hatchback_2/1(SELF_Ford_Fiesta_Hatchback_2)
  Ford_Focus_Stationwagon_1/1(STATE_Ford_Focus_Stationwagon_1_bus) -> STATE_Ford_Focus_Stationwagon_1_bus/1(STATE_Ford_Focus_Stationwagon_1_bus)
  SELF_Ford_Focus_Stationwagon_1/1(SELF_Ford_Focus_Stationwagon_1) -> Ford_Focus_Stationwagon_1/1(SELF_Ford_Focus_Stationwagon_1)
  Lexus_GS_450h_F_Sport_Sedan_1/1(STATE_Lexus_GS_450h_F_Sport_Sedan_1_bus) -> STATE_Lexus_GS_450h_F_Sport_Sedan_1_bus/1(STATE_Lexus_GS_450h_F_Sport_Sedan_1_bus)
  SELF_Lexus_GS_450h_F_Sport_Sedan_1/1(SELF_Lexus_GS_450h_F_Sport_Sedan_1) -> Lexus_GS_450h_F_Sport_Sedan_1/1(SELF_Lexus_GS_450h_F_Sport_Sedan_1)
  Lexus_LS_600h_F_Sport_1/1(STATE_Lexus_LS_600h_F_Sport_1_bus) -> STATE_Lexus_LS_600h_F_Sport_1_bus/1(STATE_Lexus_LS_600h_F_Sport_1_bus)
  SELF_Lexus_LS_600h_F_Sport_1/1(SELF_Lexus_LS_600h_F_Sport_1) -> Lexus_LS_600h_F_Sport_1/1(SELF_Lexus_LS_600h_F_Sport_1)
  Mazda_RX8_Coupe_1/1(STATE_Mazda_RX8_Coupe_1_bus) -> STATE_Mazda_RX8_Coupe_1_bus/1(STATE_Mazda_RX8_Coupe_1_bus)
  SELF_Mazda_RX8_Coupe_1/1(SELF_Mazda_RX8_Coupe_1) -> Mazda_RX8_Coupe_1/1(SELF_Mazda_RX8_Coupe_1)
  Roewe_550_S_Sedan_1/1(STATE_Roewe_550_S_Sedan_1_bus) -> STATE_Roewe_550_S_Sedan_1_bus/1(STATE_Roewe_550_S_Sedan_1_bus)
  SELF_Roewe_550_S_Sedan_1/1(SELF_Roewe_550_S_Sedan_1) -> Roewe_550_S_Sedan_1/1(SELF_Roewe_550_S_Sedan_1)
  Toyota_Previa_MPV_1/1(STATE_Toyota_Previa_MPV_1_bus) -> STATE_Toyota_Previa_MPV_1_bus/1(STATE_Toyota_Previa_MPV_1_bus)
  SELF_Toyota_Previa_MPV_1/1(SELF_Toyota_Previa_MPV_1) -> Toyota_Previa_MPV_1/1(SELF_Toyota_Previa_MPV_1)
  Toyota_Prius_Sedan_1/1(STATE_Toyota_Prius_Sedan_1_bus) -> STATE_Toyota_Prius_Sedan_1_bus/1(STATE_Toyota_Prius_Sedan_1_bus)
  SELF_Toyota_Prius_Sedan_1/1(SELF_Toyota_Prius_Sedan_1) -> Toyota_Prius_Sedan_1/1(SELF_Toyota_Prius_Sedan_1)
  Toyota_Yaris_Hatchback_1/1(STATE_Toyota_Yaris_Hatchback_1_bus) -> STATE_Toyota_Yaris_Hatchback_1_bus/1(STATE_Toyota_Yaris_Hatchback_1_bus)
  SELF_Toyota_Yaris_Hatchback_1/1(SELF_Toyota_Yaris_Hatchback_1) -> Toyota_Yaris_Hatchback_1/1(SELF_Toyota_Yaris_Hatchback_1)
  Wuling_Hongguang_1/1(STATE_Wuling_Hongguang_1_bus) -> STATE_Wuling_Hongguang_1_bus/1(STATE_Wuling_Hongguang_1_bus)
  SELF_Wuling_Hongguang_1/1(SELF_Wuling_Hongguang_1) -> Wuling_Hongguang_1/1(SELF_Wuling_Hongguang_1)
  Toyota_Yaris_Hatchback_2/1(STATE_Toyota_Yaris_Hatchback_2_bus) -> STATE_Toyota_Yaris_Hatchback_2_bus/1(STATE_Toyota_Yaris_Hatchback_2_bus)
  SELF_Toyota_Yaris_Hatchback_2/1(SELF_Toyota_Yaris_Hatchback_2) -> Toyota_Yaris_Hatchback_2/1(SELF_Toyota_Yaris_Hatchback_2)
  Citroen_C3_Hatchback_3/1(STATE_Citroen_C3_Hatchback_3_bus) -> STATE_Citroen_C3_Hatchback_3_bus/1(STATE_Citroen_C3_Hatchback_3_bus)
  SELF_Citroen_C3_Hatchback_3/1(SELF_Citroen_C3_Hatchback_3) -> Citroen_C3_Hatchback_3/1(SELF_Citroen_C3_Hatchback_3)
  Audi_A3_2/1(STATE_Audi_A3_2_bus) -> STATE_Audi_A3_2_bus/1(STATE_Audi_A3_2_bus)
  SELF_Audi_A3_2/1(SELF_Audi_A3_2) -> Audi_A3_2/1(SELF_Audi_A3_2)
  Sports_Bike_wDriver_2/1(STATE_Sports_Bike_wDriver_2_bus) -> STATE_Sports_Bike_wDriver_2_bus/1(STATE_Sports_Bike_wDriver_2_bus)
  SELF_Sports_Bike_wDriver_2/1(SELF_Sports_Bike_wDriver_2) -> Sports_Bike_wDriver_2/1(SELF_Sports_Bike_wDriver_2)
  Sports_Bike_wDriver_3/1(STATE_Sports_Bike_wDriver_3_bus) -> STATE_Sports_Bike_wDriver_3_bus/1(STATE_Sports_Bike_wDriver_3_bus)
  SELF_Sports_Bike_wDriver_3/1(SELF_Sports_Bike_wDriver_3) -> Sports_Bike_wDriver_3/1(SELF_Sports_Bike_wDriver_3)
  Honda_Pan_European_Motorcycle_With_Driver_2/1(STATE_Honda_Pan_European_Motorcycle_With_Driver_2_bus) -> STATE_Honda_Pan_European_Motorcycle_With_Driver_2_bus/1(STATE_Honda_Pan_European_Motorcycle_With_Driver_2_bus)
  SELF_Honda_Pan_European_Motorcycle_With_Driver_2/1(SELF_Honda_Pan_European_Motorcycle_With_Driver_2) -> Honda_Pan_European_Motorcycle_With_Driver_2/1(SELF_Honda_Pan_European_Motorcycle_With_Driver_2)
  Male_CyclingCyclist_1/1(STATE_Male_CyclingCyclist_1_bus) -> STATE_Male_CyclingCyclist_1_bus/1(STATE_Male_CyclingCyclist_1_bus)
  Male_CyclingCyclist_1/2(ANIM_Male_CyclingCyclist_1) -> ANIM_Male_CyclingCyclist_1/1(ANIM_Male_CyclingCyclist_1)
  SELF_Male_CyclingCyclist_1/1(SELF_Male_CyclingCyclist_1) -> Male_CyclingCyclist_1/1(SELF_Male_CyclingCyclist_1)
  Male_CyclingCyclist_2/1(STATE_Male_CyclingCyclist_2_bus) -> STATE_Male_CyclingCyclist_2_bus/1(STATE_Male_CyclingCyclist_2_bus)
  Male_CyclingCyclist_2/2(ANIM_Male_CyclingCyclist_2) -> ANIM_Male_CyclingCyclist_2/1(ANIM_Male_CyclingCyclist_2)
  SELF_Male_CyclingCyclist_2/1(SELF_Male_CyclingCyclist_2) -> Male_CyclingCyclist_2/1(SELF_Male_CyclingCyclist_2)
  Male_CyclingCyclist_3/1(STATE_Male_CyclingCyclist_3_bus) -> STATE_Male_CyclingCyclist_3_bus/1(STATE_Male_CyclingCyclist_3_bus)
  Male_CyclingCyclist_3/2(ANIM_Male_CyclingCyclist_3) -> ANIM_Male_CyclingCyclist_3/1(ANIM_Male_CyclingCyclist_3)
  SELF_Male_CyclingCyclist_3/1(SELF_Male_CyclingCyclist_3) -> Male_CyclingCyclist_3/1(SELF_Male_CyclingCyclist_3)
  Male_CyclingCyclist_4/1(STATE_Male_CyclingCyclist_4_bus) -> STATE_Male_CyclingCyclist_4_bus/1(STATE_Male_CyclingCyclist_4_bus)
  Male_CyclingCyclist_4/2(ANIM_Male_CyclingCyclist_4) -> ANIM_Male_CyclingCyclist_4/1(ANIM_Male_CyclingCyclist_4)
  SELF_Male_CyclingCyclist_4/1(SELF_Male_CyclingCyclist_4) -> Male_CyclingCyclist_4/1(SELF_Male_CyclingCyclist_4)
  Male_CyclingCyclist_5/1(STATE_Male_CyclingCyclist_5_bus) -> STATE_Male_CyclingCyclist_5_bus/1(STATE_Male_CyclingCyclist_5_bus)
  Male_CyclingCyclist_5/2(ANIM_Male_CyclingCyclist_5) -> ANIM_Male_CyclingCyclist_5/1(ANIM_Male_CyclingCyclist_5)
  SELF_Male_CyclingCyclist_5/1(SELF_Male_CyclingCyclist_5) -> Male_CyclingCyclist_5/1(SELF_Male_CyclingCyclist_5)
  Male_CyclingCyclist_6/1(STATE_Male_CyclingCyclist_6_bus) -> STATE_Male_CyclingCyclist_6_bus/1(STATE_Male_CyclingCyclist_6_bus)
  Male_CyclingCyclist_6/2(ANIM_Male_CyclingCyclist_6) -> ANIM_Male_CyclingCyclist_6/1(ANIM_Male_CyclingCyclist_6)
  SELF_Male_CyclingCyclist_6/1(SELF_Male_CyclingCyclist_6) -> Male_CyclingCyclist_6/1(SELF_Male_CyclingCyclist_6)
  Male_CyclingCyclist_7/1(STATE_Male_CyclingCyclist_7_bus) -> STATE_Male_CyclingCyclist_7_bus/1(STATE_Male_CyclingCyclist_7_bus)
  Male_CyclingCyclist_7/2(ANIM_Male_CyclingCyclist_7) -> ANIM_Male_CyclingCyclist_7/1(ANIM_Male_CyclingCyclist_7)
  SELF_Male_CyclingCyclist_7/1(SELF_Male_CyclingCyclist_7) -> Male_CyclingCyclist_7/1(SELF_Male_CyclingCyclist_7)
  Male_CyclingCyclist_8/1(STATE_Male_CyclingCyclist_8_bus) -> STATE_Male_CyclingCyclist_8_bus/1(STATE_Male_CyclingCyclist_8_bus)
  Male_CyclingCyclist_8/2(ANIM_Male_CyclingCyclist_8) -> ANIM_Male_CyclingCyclist_8/1(ANIM_Male_CyclingCyclist_8)
  SELF_Male_CyclingCyclist_8/1(SELF_Male_CyclingCyclist_8) -> Male_CyclingCyclist_8/1(SELF_Male_CyclingCyclist_8)
  Male_CyclingCyclist_9/1(STATE_Male_CyclingCyclist_9_bus) -> STATE_Male_CyclingCyclist_9_bus/1(STATE_Male_CyclingCyclist_9_bus)
  Male_CyclingCyclist_9/2(ANIM_Male_CyclingCyclist_9) -> ANIM_Male_CyclingCyclist_9/1(ANIM_Male_CyclingCyclist_9)
  SELF_Male_CyclingCyclist_9/1(SELF_Male_CyclingCyclist_9) -> Male_CyclingCyclist_9/1(SELF_Male_CyclingCyclist_9)
  Male_CyclingCyclist_10/1(STATE_Male_CyclingCyclist_10_bus) -> STATE_Male_CyclingCyclist_10_bus/1(STATE_Male_CyclingCyclist_10_bus)
  Male_CyclingCyclist_10/2(ANIM_Male_CyclingCyclist_10) -> ANIM_Male_CyclingCyclist_10/1(ANIM_Male_CyclingCyclist_10)
  SELF_Male_CyclingCyclist_10/1(SELF_Male_CyclingCyclist_10) -> Male_CyclingCyclist_10/1(SELF_Male_CyclingCyclist_10)
